simulink model "S12_PTR_Radiation_Core_v11"  (R2026a)
settings: Solver=FixedStepDiscrete  StopTime=90  FixedStep=0.02
undefined symbols (not defined in the file): s12_v11_model_ptr_radiation_step
settings Model: Creator=Jovi  LastModifiedBy=Jovi

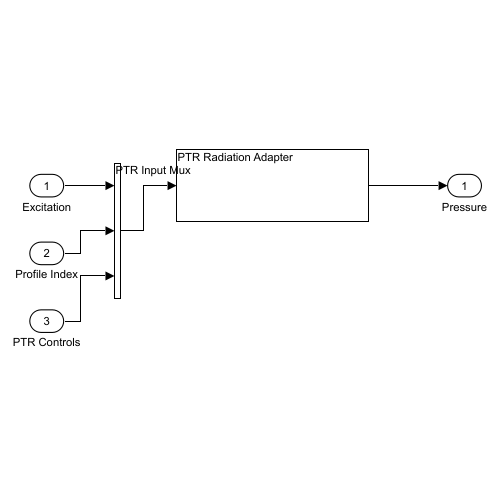
[thumbnail: Simulink's stored preview of the top-level diagram]
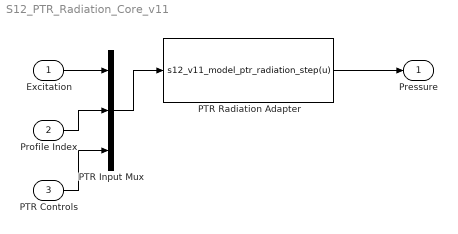
== system S12_PTR_Radiation_Core_v11 ==
  Excitation : Inport  PortDimensions=[960 1]
  Profile Index : Inport  Port=2  PortDimensions=1
  PTR Controls : Inport  Port=3  PortDimensions=[4 1]
  PTR Input Mux : Mux  Inputs=3
  PTR Radiation Adapter : MATLABFcn  MATLABFcn=s12_v11_model_ptr_radiation_step(u)  OutputDimensions=[960 1]  Output1D=off
  Pressure : Outport
  wires:
  Excitation/1 -> PTR Input Mux/1
  Profile Index/1 -> PTR Input Mux/2
  PTR Controls/1 -> PTR Input Mux/3
  PTR Input Mux/1 -> PTR Radiation Adapter/1
  PTR Radiation Adapter/1 -> Pressure/1
